simulink library "MedusaPremix"  (R2022b)
settings: Solver=VariableStepAuto  StartTime=0.0  StopTime=10.0  RelTol=1e-3
values from neighbouring files (symbols this model uses):
  PremixConfig = struct('sample_rate_in_hertz', sample_rate_in_hertz,                            'frame_size', frame_size,                            'rgain_SILENT_GAIN', rgain_SILENT_GAIN,                            'granularity', internal_granularity,                            'LR_in', LR_in, 'LR_out', LR_out,                            'CS_in', CS_in, 'CS_out', CS_out,                            'NumCenterOut' ...(+550 chars)    [MedusaPremixInit.m]
  PremixTune = MedusaPremixTuneInit(tuneFileName, headrestTuneFileName, overheadTuneFileName, MedusaParams)    [MedusaPremixInit.m]    (also in MedusaPremixTuneInit.m = load(tuneFileName))
undefined symbols (not defined in the file or in its folder): carModel, mode, MSConfig, Row
libraries: TuneVar x286, TOP x202, dspmtrx3 x146, FeaturePath x86, matrix_library x20, PooliirLib x8, Pooliir x4
(part 5 of 22)

== system MedusaPremix/PremixWithMonoSurroundAndCaeWithFadeRamper/Full Mixing Matrix_Right ==
  Audio Channel Inputs : Inport
  RST Trigger : Inport  Port=2
  SLC Request Trigger : Inport  Port=3
  In Bus Element1 : Inport  Port=4  PortName=SLC In  Element=ramp_db_per_second
  In Bus Element2 : Inport  Port=4  PortName=SLC In  Element=ramp_milliseconds
  In Bus Element : Inport  Port=4  PortName=SLC In  Element=surround_index
  SLC_NTF_check_done : Inport  Port=5
  SLC Tune In : Inport  Port=6
  Fade Request Trigger : Inport  Port=7
  Front Fade Gain : Inport  Port=8
  Back Fade Gain : Inport  Port=9
  Fade Tune In : Inport  Port=10
  Add : Sum
  Constant : Constant  OutDataTypeStr=single
  Data Store Memory1 : DataStoreMemory  DataStoreName=Premix_frameCount_Right  ReadBeforeWriteMsg=warning  WriteAfterWriteMsg=warning  WriteAfterReadMsg=warning  InitialValue=zeros(MedusaPremixConfig.LR_out,MedusaPremixConfig.LR_in)  ShowAdditionalParam=off  OutDataTypeStr=int32
  Data Store Memory2 : DataStoreMemory  DataStoreName=Premix_SLCGain_Right  ReadBeforeWriteMsg=warning  WriteAfterWriteMsg=warning  WriteAfterReadMsg=warning  InitialValue=ones(MedusaPremixConfig.LR_out,MedusaPremixConfig.LR_in)  ShowAdditionalParam=off  OutDataTypeStr=single
  Data Store Memory3 : DataStoreMemory  DataStoreName=Premix_targetGain_Right  ReadBeforeWriteMsg=warning  WriteAfterWriteMsg=warning  WriteAfterReadMsg=warning  InitialValue=ones(MedusaPremixConfig.LR_out,MedusaPremixConfig.LR_in)  ShowAdditionalParam=off  OutDataTypeStr=single
  Data Store Memory4 : DataStoreMemory  DataStoreName=Premix_currentGain_Right  ReadBeforeWriteMsg=warning  WriteAfterWriteMsg=warning  WriteAfterReadMsg=warning  InitialValue=ones(MedusaPremixConfig.LR_out,MedusaPremixConfig.LR_in)  ShowAdditionalParam=off  OutDataTypeStr=single
  Fader Downmix : Subsystem
  FeaturePath : FeaturePath/FeaturePath  FeatureName=Right  IsGroup=off  GroupNumber=-1  IsModule=off  TriggerInit=[590 34 705 141]
      settings: SourceProductName=Bose Talaria
  Matrix Multiply : Product
  Premixing : Subsystem
  Ramper : Subsystem
  Subtract : Sum  Inputs=+-
  Surround Level Control : Subsystem
  Output : Outport  VectorParamsAs1DForOutWhenUnconnected=off
  SLC_NTF_done : Outport  Port=2  VectorParamsAs1DForOutWhenUnconnected=off
  wires:
  [rampTriggerRight] -> Ramper/1(RTC Recv Trigger)
  In Bus Element1/1 -> Ramper/3(ramp rate)
  In Bus Element2/1 -> Ramper/4(ramp time)
  SLC_NTF_check_done/1 -> Ramper/5(check sequence trigger)
  [CAE_Enable] -> Fader Downmix/4(CAE_Enable)
  Front Fade Gain/1 -> Fader Downmix/1(Front Fade Gain)
  Add/1 -> Ramper/2(target gains (linear))  "Premix Matrix"
  Premixing/1(Output) -> Output/1
  Fader Downmix/2(DownmixingMatrix) -> Add/2
  SLC Tune In/1 -> Surround Level Control/4(Tuned Inputs)
  RST Trigger/1 -> Surround Level Control/1(RST Trigger)
  Ramper/1(ramping done) -> SLC_NTF_done/1
  Matrix Multiply/1 -> Add/1
  In Bus Element/1 -> Surround Level Control/3(Surround Index)
  Fade Tune In/1 -> Fader Downmix/3(Tuned Inputs)
  Fader Downmix/1(Downmix) -> Subtract/2
  Audio Channel Inputs/1 -> Premixing/1(Audio Channel Inputs)
  SLC Request Trigger/1 -> Surround Level Control/2(SLC Request Trigger)
  Fade Request Trigger/1 -> Fader Downmix/Trigger
  Back Fade Gain/1 -> Fader Downmix/2(Back Fade Gain)
  Constant/1 -> Subtract/1
  Subtract/1 -> Matrix Multiply/2  "No Downmix"
  Surround Level Control/1(Gain Out) -> Matrix Multiply/1

== system MedusaPremix/PremixWithMonoSurroundAndCaeWithFadeRamper/Generate Ramp Trigger ==
  SLCInfo : Inport
  FadeOn : Inport  Port=2
  Function-Call Split : FunctionCallSplit  IconShape=distinctive  NumOutputPorts=3  OutputPortLayout=default
  MATLAB Function : MATLAB Function  TreatAsAtomicUnit=on
  Terminator : Terminator
  tag scope: rampTriggerCS=scoped, rampTriggerLeft=scoped, rampTriggerRight=scoped
  wires:
  MATLAB Function/1(rampOn) -> Terminator/1
  SLCInfo/1 -> MATLAB Function/1(SLC_On)
  FadeOn/1 -> MATLAB Function/2(Fade_On)
  Function-Call Split/2 -> [rampTriggerCS]
  Function-Call Split/3 -> [rampTriggerRight]
  Function-Call Split/1 -> [rampTriggerLeft]
  MATLAB Function/2(ramp()) -> Function-Call Split/1

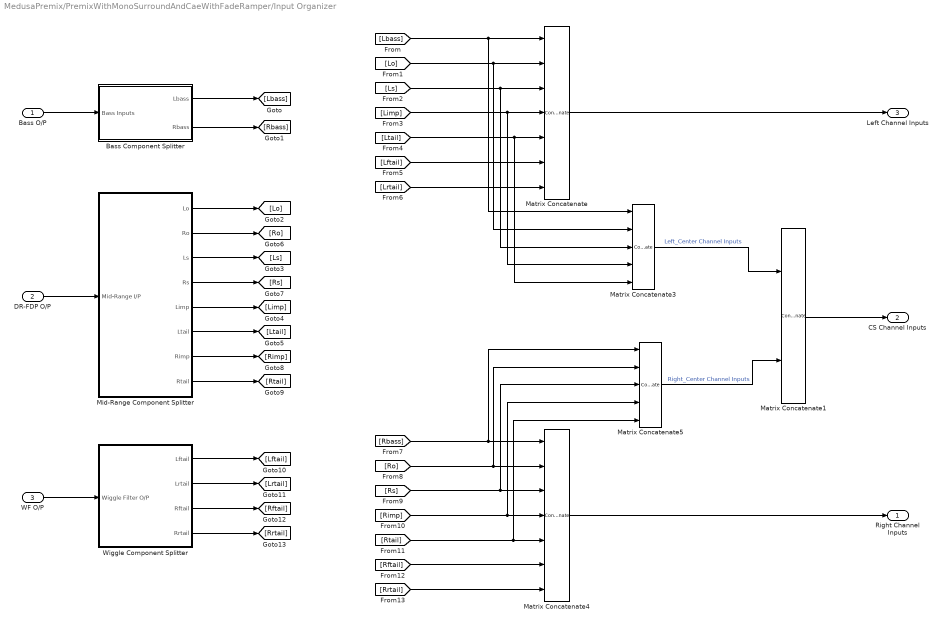
== system MedusaPremix/PremixWithMonoSurroundAndCaeWithFadeRamper/Input Organizer ==
  Bass O/P : Inport
  DR-FDP O/P : Inport  Port=2
  WF O/P : Inport  Port=3
  Bass Component Splitter : Subsystem
  Matrix Concatenate : Concatenate  NumInputs=7  Mode=Multidimensional array  ConcatenateDimension=2
  Matrix Concatenate1 : Concatenate  Mode=Multidimensional array  ConcatenateDimension=2
  Matrix Concatenate3 : Concatenate  NumInputs=5  Mode=Multidimensional array  ConcatenateDimension=2
  Matrix Concatenate4 : Concatenate  NumInputs=7  Mode=Multidimensional array  ConcatenateDimension=2
  Matrix Concatenate5 : Concatenate  NumInputs=5  Mode=Multidimensional array  ConcatenateDimension=2
  Mid-Range Component Splitter : Subsystem
  Wiggle Component Splitter : Subsystem
  Right Channel Inputs : Outport  VectorParamsAs1DForOutWhenUnconnected=off
  CS Channel Inputs : Outport  Port=2  VectorParamsAs1DForOutWhenUnconnected=off
  Left Channel Inputs : Outport  Port=3  VectorParamsAs1DForOutWhenUnconnected=off
  wires:
  Matrix Concatenate4/1 -> Right Channel Inputs/1
  [Ltail] -> Matrix Concatenate3/5, Matrix Concatenate/5
  Matrix Concatenate5/1 -> Matrix Concatenate1/2  "Right_Center Channel Inputs"
  [Limp] -> Matrix Concatenate3/4, Matrix Concatenate/4
  [Rimp] -> Matrix Concatenate5/4, Matrix Concatenate4/4
  [Rbass] -> Matrix Concatenate5/1, Matrix Concatenate4/1
  Matrix Concatenate1/1 -> CS Channel Inputs/1
  Wiggle Component Splitter/2(Lrtail) -> [Lrtail]
  Wiggle Component Splitter/1(Lftail) -> [Lftail]
  Bass Component Splitter/2(Rbass) -> [Rbass]
  DR-FDP O/P/1 -> Mid-Range Component Splitter/1(Mid-Range I/P)
  [Ro] -> Matrix Concatenate5/2, Matrix Concatenate4/2
  Wiggle Component Splitter/3(Rftail) -> [Rftail]
  Bass O/P/1 -> Bass Component Splitter/1(Bass Inputs)
  Matrix Concatenate/1 -> Left Channel Inputs/1
  [Lrtail] -> Matrix Concatenate/7
  [Lftail] -> Matrix Concatenate/6
  [Rs] -> Matrix Concatenate5/3, Matrix Concatenate4/3
  WF O/P/1 -> Wiggle Component Splitter/1(Wiggle Filter O/P)
  [Rtail] -> Matrix Concatenate5/5, Matrix Concatenate4/5
  [Ls] -> Matrix Concatenate3/3, Matrix Concatenate/3
  [Lbass] -> Matrix Concatenate3/1, Matrix Concatenate/1
  Matrix Concatenate3/1 -> Matrix Concatenate1/1  "Left_Center Channel Inputs"
  [Lo] -> Matrix Concatenate3/2, Matrix Concatenate/2
  Wiggle Component Splitter/4(Rrtail) -> [Rrtail]
  Mid-Range Component Splitter/1(Lo) -> [Lo]
  [Rftail] -> Matrix Concatenate4/6
  Bass Component Splitter/1(Lbass) -> [Lbass]
  [Rrtail] -> Matrix Concatenate4/7
  Mid-Range Component Splitter/2(Ro) -> [Ro]
  Mid-Range Component Splitter/3(Ls) -> [Ls]
  Mid-Range Component Splitter/4(Rs) -> [Rs]
  Mid-Range Component Splitter/5(Limp) -> [Limp]
  Mid-Range Component Splitter/6(Ltail) -> [Ltail]
  Mid-Range Component Splitter/7(Rimp) -> [Rimp]
  Mid-Range Component Splitter/8(Rtail) -> [Rtail]

== system MedusaPremix/PremixWithMonoSurroundAndCaeWithFadeRamper/Merge NTF_done ==
  SLC_NTF_done_Left : Inport
  SLC_NTF_done_CS : Inport  Port=2
  SLC_NTF_done_Right : Inport  Port=3
  Trigger : TriggerPort  TriggerType=function-call  VariantControl=Variant  PortDimensions=1
  AND : Logic  Inputs=3  IconShape=distinctive  AllPortsSameDT=off  OutDataTypeStr=boolean
  SLC_NTF_done : Outport  VectorParamsAs1DForOutWhenUnconnected=off
  wires:
  SLC_NTF_done_Right/1 -> AND/1
  SLC_NTF_done_CS/1 -> AND/2
  SLC_NTF_done_Left/1 -> AND/3
  AND/1 -> SLC_NTF_done/1

== system MedusaPremix/PremixWithMonoSurroundAndCaeWithFadeRamper/SLC Tuning ==
  Detent Level CS : Subsystem  Description="This is the premix (scalar mixing) matrix for the detent (default) level of \"surroundiness\"."
  Detent Level Left : Subsystem  Description="This is the premix (scalar mixing) matrix for the detent (default) level of \"surroundiness\"."
  Detent Level Right : Subsystem  Description="This is the premix (scalar mixing) matrix for the detent (default) level of \"surroundiness\"."
  Interpolation Method : Subsystem  Description=|
      | This controls the method used to interpolate premix coefficient matrix as the surround knob is adjusted.
      | - 0 for linear interpolation (default)
      | - 1 for db-linear interpolation
  Max Level CS : Subsystem  Description="This is the premix (scalar mixing) matrix for the maximum level of \"surroundiness\"."
  Max Level Left : Subsystem  Description="This is the premix (scalar mixing) matrix for the maximum level of \"surroundiness\"."
  Max Level Right : Subsystem  Description="This is the premix (scalar mixing) matrix for the maximum level of \"surroundiness\"."
  Min Level CS : Subsystem  Description="This is the premix (scalar mixing) matrix for the minimum level of \"surroundiness\" i.e. steroe case."
  Min Level Left : Subsystem  Description="This is the premix (scalar mixing) matrix for the minimum level of \"surroundiness\" i.e. steroe case."
  Min Level Right : Subsystem  Description="This is the premix (scalar mixing) matrix for the minimum level of \"surroundiness\" i.e. steroe case."
  Bus Element Out : Outport  VectorParamsAs1DForOutWhenUnconnected=off  PortName=SLC Tune Out  Element=Interpolation Method
  Bus Element Out1 : Outport  VectorParamsAs1DForOutWhenUnconnected=off  PortName=SLC Tune Out  Element=Min Level Left
  Bus Element Out2 : Outport  VectorParamsAs1DForOutWhenUnconnected=off  PortName=SLC Tune Out  Element=Detent Level Left
  Bus Element Out3 : Outport  VectorParamsAs1DForOutWhenUnconnected=off  PortName=SLC Tune Out  Element=Max Level Left
  Bus Element Out4 : Outport  VectorParamsAs1DForOutWhenUnconnected=off  PortName=SLC Tune Out  Element=Min Level CS
  Bus Element Out5 : Outport  VectorParamsAs1DForOutWhenUnconnected=off  PortName=SLC Tune Out  Element=Detent Level CS
  Bus Element Out6 : Outport  VectorParamsAs1DForOutWhenUnconnected=off  PortName=SLC Tune Out  Element=Max Level CS
  Bus Element Out7 : Outport  VectorParamsAs1DForOutWhenUnconnected=off  PortName=SLC Tune Out  Element=Min Level Right
  Bus Element Out8 : Outport  VectorParamsAs1DForOutWhenUnconnected=off  PortName=SLC Tune Out  Element=Detent Level Right
  Bus Element Out9 : Outport  VectorParamsAs1DForOutWhenUnconnected=off  PortName=SLC Tune Out  Element=Max Level Right
  Bus Element Out10 : Outport  VectorParamsAs1DForOutWhenUnconnected=off  PortName=SLC Tune Out  Element=Min Level Left CAE
  Bus Element Out11 : Outport  VectorParamsAs1DForOutWhenUnconnected=off  PortName=SLC Tune Out  Element=Detent Level Left CAE
  Bus Element Out12 : Outport  VectorParamsAs1DForOutWhenUnconnected=off  PortName=SLC Tune Out  Element=Max Level Left CAE
  Bus Element Out13 : Outport  VectorParamsAs1DForOutWhenUnconnected=off  PortName=SLC Tune Out  Element=Min Level CS CAE
  Bus Element Out14 : Outport  VectorParamsAs1DForOutWhenUnconnected=off  PortName=SLC Tune Out  Element=Detent Level CS CAE
  Bus Element Out15 : Outport  VectorParamsAs1DForOutWhenUnconnected=off  PortName=SLC Tune Out  Element=Max Level CS CAE
  Bus Element Out16 : Outport  VectorParamsAs1DForOutWhenUnconnected=off  PortName=SLC Tune Out  Element=Min Level Right CAE
  Bus Element Out17 : Outport  VectorParamsAs1DForOutWhenUnconnected=off  PortName=SLC Tune Out  Element=Detent Level Right CAE
  Bus Element Out18 : Outport  VectorParamsAs1DForOutWhenUnconnected=off  PortName=SLC Tune Out  Element=Max Level Right CAE
  wires:
  Min Level Left/2(Out2) -> Bus Element Out10/1
  Max Level Right/2(Out2) -> Bus Element Out18/1
  Detent Level Right/2(Out2) -> Bus Element Out17/1
  Min Level Right/2(Out2) -> Bus Element Out16/1
  Max Level CS/2(Out2) -> Bus Element Out15/1
  Detent Level CS/2(Out2) -> Bus Element Out14/1
  Min Level CS/2(Out2) -> Bus Element Out13/1
  Max Level Left/2(Out2) -> Bus Element Out12/1
  Detent Level Left/2(Out2) -> Bus Element Out11/1
  Min Level Right/1(Out1) -> Bus Element Out7/1
  Max Level Right/1(Out1) -> Bus Element Out9/1
  Detent Level Right/1(Out1) -> Bus Element Out8/1
  Detent Level CS/1(Out1) -> Bus Element Out5/1
  Min Level CS/1(Out1) -> Bus Element Out4/1
  Max Level CS/1(Out1) -> Bus Element Out6/1
  Max Level Left/1(Out1) -> Bus Element Out3/1
  Detent Level Left/1(Out1) -> Bus Element Out2/1
  Min Level Left/1(Out1) -> Bus Element Out1/1
  Interpolation Method/1(Out1) -> Bus Element Out/1

== system MedusaPremix/Premix/Fade Tuning/Backward Downmix Max ==
  TOP : TOP/TOP  TriggerInit=[440 20 585 80]  TopName=BackwardDownmixMax  DataType=single  BankNumber=0  Role=Automatic
      settings: SourceProductName=Bose Talaria
  TranslateTrigger : TuneVar/TranslateTrigger  TriggerInit=[286 -100 324 -45]
      settings: SourceProductName=Bose Talaria
  Trivial Translation : MATLAB Function  TreatAsAtomicUnit=on
  Tune Variable : TuneVar/Tune Variable  TuneName=BackwardDownmixMax  SpecifyMaxSize=off  VariableDim=1 (Row)  MaxSize=[1 1]  PackageName=mode  TunabilityNumber=1  MinValue=[0]  MaxValue=[1]  TriggerInit=[-65 25 105 75]  MaskValue=MedusaPremixTune.BackwardDownmixMax
      settings: SourceProductName=Bose Talaria
  Out1 : Outport  VectorParamsAs1DForOutWhenUnconnected=off
  wires:
  TOP/1 -> Out1/1  "BackwardDownmixMax"
  Tune Variable/1 -> Trivial Translation/1(BackwardDownmixMax)  "BackwardDownmixMax"
  Trivial Translation/1(TOP) -> TOP/1
  TranslateTrigger/1 -> Trivial Translation/Trigger

== system MedusaPremix/Premix/Fade Tuning/Backward Downmix Threshold ==
  TOP : TOP/TOP  TriggerInit=[440 20 585 80]  TopName=BackwardDownmixThreshold  DataType=single  BankNumber=0  Role=Automatic
      settings: SourceProductName=Bose Talaria
  TranslateTrigger : TuneVar/TranslateTrigger  TriggerInit=[306 -100 344 -45]
      settings: SourceProductName=Bose Talaria
  Trivial Translation : MATLAB Function  TreatAsAtomicUnit=on
  Tune Variable : TuneVar/Tune Variable  TuneName=BackwardDownmixThreshold  SpecifyMaxSize=off  VariableDim=1 (Row)  MaxSize=[1 1]  PackageName=mode  TunabilityNumber=1  MinValue=[0]  MaxValue=[1]  TriggerInit=[-75 25 95 75]  MaskValue=MedusaPremixTune.BackwardDownmixThreshold
      settings: SourceProductName=Bose Talaria
  Out1 : Outport  VectorParamsAs1DForOutWhenUnconnected=off
  wires:
  TOP/1 -> Out1/1  "BackwardDownmixThreshold"
  Tune Variable/1 -> Trivial Translation/1(BackwardDownmixThreshold)  "BackwardDownmixThreshold"
  Trivial Translation/1(TOP) -> TOP/1
  TranslateTrigger/1 -> Trivial Translation/Trigger

== system MedusaPremix/Premix/Fade Tuning/Downmix Weights CS ==
  TOP : TOP/TOP  TriggerInit=[440 20 585 80]  TopName=DownmixWeights_CS  DataType=single  BankNumber=0  Role=Automatic
      settings: SourceProductName=Bose Talaria
  TranslateTrigger : TuneVar/TranslateTrigger  TriggerInit=[256 -100 294 -45]
      settings: SourceProductName=Bose Talaria
  Trivial Translation : MATLAB Function  TreatAsAtomicUnit=on
  Tune Variable : TuneVar/Tune Variable  TuneName=DownmixWeights_CS  SpecifyMaxSize=off  VariableDim=1 (Row)  MaxSize=[1 1]  PackageName=mode  TunabilityNumber=1  MinValue=[0]  MaxValue=[1]  TriggerInit=[-85 25 85 75]  MaskValue=MedusaPremixTune.downmix_wts_CS
      settings: SourceProductName=Bose Talaria
  Out1 : Outport  VectorParamsAs1DForOutWhenUnconnected=off
  wires:
  TOP/1 -> Out1/1  "DownmixWeights_CS"
  Tune Variable/1 -> Trivial Translation/1(downmix_wts_CS)  "DownmixWeights_CS"
  Trivial Translation/1(TOP) -> TOP/1
  TranslateTrigger/1 -> Trivial Translation/Trigger

== system MedusaPremix/Premix/Fade Tuning/Downmix Weights Left ==
  TOP : TOP/TOP  TriggerInit=[440 20 585 80]  TopName=DownmixWeights_Left  DataType=single  BankNumber=0  Role=Automatic
      settings: SourceProductName=Bose Talaria
  TranslateTrigger : TuneVar/TranslateTrigger  TriggerInit=[266 -100 304 -45]
      settings: SourceProductName=Bose Talaria
  Trivial Translation : MATLAB Function  TreatAsAtomicUnit=on
  Tune Variable : TuneVar/Tune Variable  TuneName=DownmixWeights_Left  SpecifyMaxSize=off  VariableDim=1 (Row)  MaxSize=[1 1]  PackageName=mode  TunabilityNumber=1  MinValue=[0]  MaxValue=[1]  TriggerInit=[-80 25 90 75]  MaskValue=MedusaPremixTune.downmix_wts_Left
      settings: SourceProductName=Bose Talaria
  Out1 : Outport  VectorParamsAs1DForOutWhenUnconnected=off
  wires:
  TOP/1 -> Out1/1  "DownmixWeights_Left"
  Tune Variable/1 -> Trivial Translation/1(downmix_wts_Left)  "DownmixWeights_Left"
  Trivial Translation/1(TOP) -> TOP/1
  TranslateTrigger/1 -> Trivial Translation/Trigger

== system MedusaPremix/Premix/Fade Tuning/Downmix Weights Right ==
  TOP : TOP/TOP  TriggerInit=[475 20 620 80]  TopName=DownmixWeights_Right  DataType=single  BankNumber=0  Role=Automatic
      settings: SourceProductName=Bose Talaria
  TranslateTrigger : TuneVar/TranslateTrigger  TriggerInit=[306 -100 344 -45]
      settings: SourceProductName=Bose Talaria
  Trivial Translation : MATLAB Function  TreatAsAtomicUnit=on
  Tune Variable : TuneVar/Tune Variable  TuneName=DownmixWeights_Right  SpecifyMaxSize=off  VariableDim=1 (Row)  MaxSize=[1 1]  PackageName=mode  TunabilityNumber=1  MinValue=[0]  MaxValue=[1]  TriggerInit=[-40 25 130 75]  MaskValue=MedusaPremixTune.downmix_wts_Right
      settings: SourceProductName=Bose Talaria
  Out1 : Outport  VectorParamsAs1DForOutWhenUnconnected=off
  wires:
  TOP/1 -> Out1/1  "DownmixWeights_Right"
  Tune Variable/1 -> Trivial Translation/1(downmix_wts_Right)  "DownmixWeights_Right"
  Trivial Translation/1(TOP) -> TOP/1
  TranslateTrigger/1 -> Trivial Translation/Trigger

== system MedusaPremix/Premix/Fade Tuning/Forward Downmix Threshold ==
  TOP : TOP/TOP  TriggerInit=[440 20 585 80]  TopName=ForwardDownmixThreshold  DataType=single  BankNumber=0  Role=Automatic
      settings: SourceProductName=Bose Talaria
  TranslateTrigger : TuneVar/TranslateTrigger  TriggerInit=[291 -100 329 -45]
      settings: SourceProductName=Bose Talaria
  Trivial Translation : MATLAB Function  TreatAsAtomicUnit=on
  Tune Variable : TuneVar/Tune Variable  TuneName=ForwardDownmixThreshold  SpecifyMaxSize=off  VariableDim=1 (Row)  MaxSize=[1 1]  PackageName=mode  TunabilityNumber=1  MinValue=[0]  MaxValue=[1]  TriggerInit=[-80 25 90 75]  MaskValue=MedusaPremixTune.ForwardDownmixThreshold
      settings: SourceProductName=Bose Talaria
  Out1 : Outport  VectorParamsAs1DForOutWhenUnconnected=off
  wires:
  TOP/1 -> Out1/1  "ForwardDownmixThreshold"
  Tune Variable/1 -> Trivial Translation/1(ForwardDownmixThreshold)  "ForwardDownmixThreshold"
  Trivial Translation/1(TOP) -> TOP/1
  TranslateTrigger/1 -> Trivial Translation/Trigger

== system MedusaPremix/Premix/Fade Tuning/Foward Downmix Max ==
  TOP : TOP/TOP  TriggerInit=[440 20 585 80]  TopName=ForwardDownmixMax  DataType=single  BankNumber=0  Role=Automatic
      settings: SourceProductName=Bose Talaria
  TranslateTrigger : TuneVar/TranslateTrigger  TriggerInit=[286 -100 324 -45]
      settings: SourceProductName=Bose Talaria
  Trivial Translation : MATLAB Function  TreatAsAtomicUnit=on
  Tune Variable : TuneVar/Tune Variable  TuneName=ForwardDownmixMax  SpecifyMaxSize=off  VariableDim=1 (Row)  MaxSize=[1 1]  PackageName=mode  TunabilityNumber=1  MinValue=[0]  MaxValue=[1]  TriggerInit=[-70 25 100 75]  MaskValue=MedusaPremixTune.ForwardDownmixMax
      settings: SourceProductName=Bose Talaria
  Out1 : Outport  VectorParamsAs1DForOutWhenUnconnected=off
  wires:
  TOP/1 -> Out1/1  "ForwardDownmixMax"
  Tune Variable/1 -> Trivial Translation/1(ForwardDownmixMax)  "ForwardDownmixMax"
  Trivial Translation/1(TOP) -> TOP/1
  TranslateTrigger/1 -> Trivial Translation/Trigger

== system MedusaPremix/Premix/Full Mixing Matrix_Center Surround/Fader Downmix ==
  note: downmix
  Front Fade Gain : Inport
  Back Fade Gain : Inport  Port=2
  In Bus Element : Inport  Port=3  PortName=Tuned Inputs  Element=Forward Downmix Threshold
  In Bus Element1 : Inport  Port=3  PortName=Tuned Inputs  Element=Forward Downmix Max
  In Bus Element2 : Inport  Port=3  PortName=Tuned Inputs  Element=Backward Downmix Threshold
  In Bus Element3 : Inport  Port=3  PortName=Tuned Inputs  Element=Backward Downmix Max
  In Bus Element4 : Inport  Port=3  PortName=Tuned Inputs  Element=Downmix Weights CS
  Trigger : TriggerPort  TriggerType=function-call  VariantControl=Variant  PortDimensions=1
  Fading Backward : Subsystem  TreatAsAtomicUnit=on
  Fading Forward : Subsystem  TreatAsAtomicUnit=on
  FeaturePath : FeaturePath/FeaturePath  FeatureName=Fade  IsGroup=off  GroupNumber=-1  DeclarePackages=off  PackageNames=mode,carModel  IsToolGroup=off  TriggerInit=[920 94 1035 201]
      settings: SourceProductName=Bose Talaria
  If : If  NumInputs=2  IfExpression=u1 >= u2
  Matrix Multiply : Product
  Merge : Merge
  Downmix : Outport  VectorParamsAs1DForOutWhenUnconnected=off
  DownmixingMatrix : Outport  Port=2  VectorParamsAs1DForOutWhenUnconnected=off
  wires:
  If/1 -> Fading Forward/Action
  Fading Backward/1(downmix) -> Merge/2
  Front Fade Gain/1 -> If/1, Fading Backward/1(frontFadeGain)
  Merge/1 -> Matrix Multiply/1, Downmix/1
  Back Fade Gain/1 -> Fading Forward/1(backFadeGain), If/2
  Matrix Multiply/1 -> DownmixingMatrix/1
  Fading Forward/1(downmix) -> Merge/1
  If/2 -> Fading Backward/Action
  In Bus Element/1 -> Fading Forward/2(forwardDownmixThreshold)
  In Bus Element1/1 -> Fading Forward/3(forwardDownmixMax)
  In Bus Element2/1 -> Fading Backward/2(backwardDownmixThreshold)
  In Bus Element3/1 -> Fading Backward/3(backwardDownmixMax)
  In Bus Element4/1 -> Matrix Multiply/2

== system MedusaPremix/Premix/Full Mixing Matrix_Center Surround/Premixing ==
  Audio Channel Inputs : Inport
  Target Gain : Inport  Port=2
  Matrix Multiply1 : Product  Multiplication=Matrix(*)
  Transpose1 : Math  Operator=transpose  SignedPower=on
  Output : Outport  VectorParamsAs1DForOutWhenUnconnected=off
  wires:
  Transpose1/1 -> Matrix Multiply1/2
  Target Gain/1 -> Transpose1/1
  Audio Channel Inputs/1 -> Matrix Multiply1/1
  Matrix Multiply1/1 -> Output/1

== system MedusaPremix/Premix/Full Mixing Matrix_Center Surround/Surround Level Control ==
  RST Trigger : Inport
  SLC Request Trigger : Inport  Port=2
  In Bus Element : Inport  Port=3  PortName=Control Inputs  Element=surround_index
  In Bus Element1 : Inport  Port=3  PortName=Control Inputs  Element=ramp_db_per_second
  In Bus Element2 : Inport  Port=3  PortName=Control Inputs  Element=ramp_milliseconds
  Check Done : Inport  Port=4
  In Bus Element3 : Inport  Port=5  PortName=Tuned Inputs  Element=Min Level CS
  In Bus Element4 : Inport  Port=5  PortName=Tuned Inputs  Element=Detent Level CS
  In Bus Element5 : Inport  Port=5  PortName=Tuned Inputs  Element=Max Level CS
  In Bus Element6 : Inport  Port=5  PortName=Tuned Inputs  Element=Interpolation Method
  Data Store Memory3 : DataStoreMemory  DataStoreName=Premix_targetGain_CS  ReadBeforeWriteMsg=warning  WriteAfterWriteMsg=warning  WriteAfterReadMsg=warning  InitialValue=1e-5*ones(MedusaPremixConfig.CS_out,MedusaPremixConfig.CS_in)  ShowAdditionalParam=off  OutDataTypeStr=single
  Data Store Memory4 : DataStoreMemory  DataStoreName=Premix_currentGain_CS  ReadBeforeWriteMsg=warning  WriteAfterWriteMsg=warning  WriteAfterReadMsg=warning  InitialValue=1e-5*ones(MedusaPremixConfig.CS_out,MedusaPremixConfig.CS_in)  ShowAdditionalParam=off  OutDataTypeStr=single
  Data Store Read1 : DataStoreRead  DataStoreName=Premix_currentGain_CS  IndexOptions=Index vector (dialog)  Indices=1  OutputSizes=1
  FeaturePath : FeaturePath/FeaturePath  FeatureName=SLC  IsGroup=off  GroupNumber=-1  DeclarePackages=off  PackageNames=mode,carModel  IsToolGroup=off  TriggerInit=[955 334 1070 441]
      settings: SourceProductName=Bose Talaria
  Function-Call Split : FunctionCallSplit  IconShape=distinctive  NumOutputPorts=2
  Initialization and RMDL : MATLAB Function  TreatAsAtomicUnit=on
  Ramper : Subsystem
  Target Gain Computation : MATLAB Function  TreatAsAtomicUnit=on
  Gain Out : Outport  VectorParamsAs1DForOutWhenUnconnected=off
  Ramping Done : Outport  Port=2  VectorParamsAs1DForOutWhenUnconnected=off
  wires:
  Data Store Read1/1 -> Gain Out/1
  RST Trigger/1 -> Initialization and RMDL/Trigger
  Check Done/1 -> Ramper/5(check sequence trigger)
  Target Gain Computation/1(gain_out) -> Ramper/2(target gains (linear))
  Function-Call Split/1 -> Target Gain Computation/Trigger
  Function-Call Split/2 -> Ramper/1(RTC Recv Trigger)
  SLC Request Trigger/1 -> Function-Call Split/1
  Ramper/1(ramping done) -> Ramping Done/1
  In Bus Element5/1 -> Initialization and RMDL/3(maxGain_CS), Target Gain Computation/3(maxGain_CS)
  In Bus Element6/1 -> Initialization and RMDL/4(interpolation_method), Target Gain Computation/4(interpolation_method)
  In Bus Element3/1 -> Initialization and RMDL/1(minGain_CS), Target Gain Computation/1(minGain_CS)
  In Bus Element4/1 -> Initialization and RMDL/2(detentGain_CS), Target Gain Computation/2(detentGain_CS)
  In Bus Element2/1 -> Ramper/4(ramp time)
  In Bus Element1/1 -> Ramper/3(ramp rate)
  In Bus Element/1 -> Initialization and RMDL/5(surr_level), Target Gain Computation/5(surr_level)

== system MedusaPremix/Premix/Full Mixing Matrix_Left/Fader Downmix ==
  note: downmix
  Front Fade Gain : Inport
  Back Fade Gain : Inport  Port=2
  In Bus Element : Inport  Port=3  PortName=Tuned Inputs  Element=Forward Downmix Threshold
  In Bus Element1 : Inport  Port=3  PortName=Tuned Inputs  Element=Forward Downmix Max
  In Bus Element2 : Inport  Port=3  PortName=Tuned Inputs  Element=Backward Downmix Threshold
  In Bus Element3 : Inport  Port=3  PortName=Tuned Inputs  Element=Backward Downmix Max
  In Bus Element4 : Inport  Port=3  PortName=Tuned Inputs  Element=Downmix Weights Left
  Trigger : TriggerPort  TriggerType=function-call  VariantControl=Variant  PortDimensions=1
  Fading Backward : Subsystem  TreatAsAtomicUnit=on
  Fading Forward : Subsystem  TreatAsAtomicUnit=on
  FeaturePath : FeaturePath/FeaturePath  FeatureName=Fade  IsGroup=off  GroupNumber=-1  DeclarePackages=off  PackageNames=mode,carModel  IsToolGroup=off  TriggerInit=[875 94 990 201]
      settings: SourceProductName=Bose Talaria
  If : If  NumInputs=2  IfExpression=u1 >= u2
  Matrix Multiply : Product
  Merge : Merge
  Downmix : Outport  VectorParamsAs1DForOutWhenUnconnected=off
  DownmixingMatrix : Outport  Port=2  VectorParamsAs1DForOutWhenUnconnected=off
  wires:
  If/1 -> Fading Forward/Action
  Fading Backward/1(downmix) -> Merge/2
  Front Fade Gain/1 -> If/1, Fading Backward/1(frontFadeGain)
  Merge/1 -> Matrix Multiply/1, Downmix/1
  Back Fade Gain/1 -> Fading Forward/1(backFadeGain), If/2
  Matrix Multiply/1 -> DownmixingMatrix/1
  Fading Forward/1(downmix) -> Merge/1
  If/2 -> Fading Backward/Action
  In Bus Element/1 -> Fading Forward/2(forwardDownmixThreshold)
  In Bus Element1/1 -> Fading Forward/3(forwardDownmixMax)
  In Bus Element2/1 -> Fading Backward/2(backwardDownmixThreshold)
  In Bus Element3/1 -> Fading Backward/3(backwardDownmixMax)
  In Bus Element4/1 -> Matrix Multiply/2

== system MedusaPremix/Premix/Full Mixing Matrix_Left/Premixing ==
  Audio Channel Inputs : Inport
  Target Gain : Inport  Port=2
  Matrix Multiply1 : Product  Multiplication=Matrix(*)
  Transpose1 : Math  Operator=transpose  SignedPower=on
  Output : Outport  VectorParamsAs1DForOutWhenUnconnected=off
  wires:
  Transpose1/1 -> Matrix Multiply1/2
  Target Gain/1 -> Transpose1/1
  Audio Channel Inputs/1 -> Matrix Multiply1/1
  Matrix Multiply1/1 -> Output/1

== system MedusaPremix/Premix/Full Mixing Matrix_Left/Surround Level Control ==
  RST Trigger : Inport
  SLC Request Trigger : Inport  Port=2
  In Bus Element : Inport  Port=3  PortName=Control Inputs  Element=surround_index
  In Bus Element1 : Inport  Port=3  PortName=Control Inputs  Element=ramp_db_per_second
  In Bus Element2 : Inport  Port=3  PortName=Control Inputs  Element=ramp_milliseconds
  Check Done : Inport  Port=4
  In Bus Element3 : Inport  Port=5  PortName=Tuned Inputs  Element=Min Level Left
  In Bus Element4 : Inport  Port=5  PortName=Tuned Inputs  Element=Detent Level Left
  In Bus Element5 : Inport  Port=5  PortName=Tuned Inputs  Element=Max Level Left
  In Bus Element6 : Inport  Port=5  PortName=Tuned Inputs  Element=Interpolation Method
  Data Store Memory3 : DataStoreMemory  DataStoreName=Premix_targetGain_Left  ReadBeforeWriteMsg=warning  WriteAfterWriteMsg=warning  WriteAfterReadMsg=warning  InitialValue=1e-5*ones(MedusaPremixConfig.LR_out,MedusaPremixConfig.LR_in)  ShowAdditionalParam=off  OutDataTypeStr=single
  Data Store Memory4 : DataStoreMemory  DataStoreName=Premix_currentGain_Left  ReadBeforeWriteMsg=warning  WriteAfterWriteMsg=warning  WriteAfterReadMsg=warning  InitialValue=1e-5*ones(MedusaPremixConfig.LR_out,MedusaPremixConfig.LR_in)  ShowAdditionalParam=off  OutDataTypeStr=single
  Data Store Read1 : DataStoreRead  DataStoreName=Premix_currentGain_Left  IndexOptions=Index vector (dialog)  Indices=1  OutputSizes=1
  FeaturePath : FeaturePath/FeaturePath  FeatureName=SLC  IsGroup=off  GroupNumber=-1  DeclarePackages=off  PackageNames=mode,carModel  IsToolGroup=off  TriggerInit=[955 334 1070 441]
      settings: SourceProductName=Bose Talaria
  Function-Call Split : FunctionCallSplit  IconShape=distinctive  NumOutputPorts=2
  Initialization and RMDL : MATLAB Function  TreatAsAtomicUnit=on
  Ramper : Subsystem
  Target Gain Computation : MATLAB Function  TreatAsAtomicUnit=on
  Gain Out : Outport  VectorParamsAs1DForOutWhenUnconnected=off
  Ramping Done : Outport  Port=2  VectorParamsAs1DForOutWhenUnconnected=off
  wires:
  In Bus Element2/1 -> Ramper/4(ramp time)
  In Bus Element1/1 -> Ramper/3(ramp rate)
  In Bus Element/1 -> Target Gain Computation/5(surr_level), Initialization and RMDL/5(surr_level)
  Data Store Read1/1 -> Gain Out/1
  RST Trigger/1 -> Initialization and RMDL/Trigger
  Check Done/1 -> Ramper/5(check sequence trigger)
  Target Gain Computation/1(gain_out) -> Ramper/2(target gains (linear))
  Function-Call Split/1 -> Target Gain Computation/Trigger
  Function-Call Split/2 -> Ramper/1(RTC Recv Trigger)
  SLC Request Trigger/1 -> Function-Call Split/1
  Ramper/1(ramping done) -> Ramping Done/1
  In Bus Element5/1 -> Target Gain Computation/3(maxGain_Left), Initialization and RMDL/3(maxGain_Left)
  In Bus Element6/1 -> Target Gain Computation/4(interpolation_method), Initialization and RMDL/4(interpolation_method)
  In Bus Element3/1 -> Target Gain Computation/1(minGain_Left), Initialization and RMDL/1(minGain_Left)
  In Bus Element4/1 -> Initialization and RMDL/2(detentGain_Left), Target Gain Computation/2(detentGain_Left)

== system MedusaPremix/Premix/Full Mixing Matrix_Right/Fader Downmix ==
  note: downmix
  Front Fade Gain : Inport
  Back Fade Gain : Inport  Port=2
  In Bus Element : Inport  Port=3  PortName=Tuned Inputs  Element=Forward Downmix Threshold
  In Bus Element1 : Inport  Port=3  PortName=Tuned Inputs  Element=Forward Downmix Max
  In Bus Element2 : Inport  Port=3  PortName=Tuned Inputs  Element=Backward Downmix Threshold
  In Bus Element3 : Inport  Port=3  PortName=Tuned Inputs  Element=Backward Downmix Max
  In Bus Element4 : Inport  Port=3  PortName=Tuned Inputs  Element=Downmix Weights Right
  Trigger : TriggerPort  TriggerType=function-call  VariantControl=Variant  PortDimensions=1
  Fading Backward : Subsystem  TreatAsAtomicUnit=on
  Fading Forward : Subsystem  TreatAsAtomicUnit=on
  FeaturePath : FeaturePath/FeaturePath  FeatureName=Fade  IsGroup=off  GroupNumber=-1  DeclarePackages=off  PackageNames=mode,carModel  IsToolGroup=off  TriggerInit=[875 94 990 201]
      settings: SourceProductName=Bose Talaria
  If : If  NumInputs=2  IfExpression=u1 >= u2
  Matrix Multiply : Product
  Merge : Merge
  Downmix : Outport  VectorParamsAs1DForOutWhenUnconnected=off
  DownmixingMatrix : Outport  Port=2  VectorParamsAs1DForOutWhenUnconnected=off
  wires:
  If/1 -> Fading Forward/Action
  Fading Backward/1(downmix) -> Merge/2
  Front Fade Gain/1 -> If/1, Fading Backward/1(frontFadeGain)
  Merge/1 -> Matrix Multiply/1, Downmix/1
  Back Fade Gain/1 -> Fading Forward/1(backFadeGain), If/2
  Matrix Multiply/1 -> DownmixingMatrix/1
  Fading Forward/1(downmix) -> Merge/1
  If/2 -> Fading Backward/Action
  In Bus Element/1 -> Fading Forward/2(forwardDownmixThreshold)
  In Bus Element1/1 -> Fading Forward/3(forwardDownmixMax)
  In Bus Element2/1 -> Fading Backward/2(backwardDownmixThreshold)
  In Bus Element3/1 -> Fading Backward/3(backwardDownmixMax)
  In Bus Element4/1 -> Matrix Multiply/2

== system MedusaPremix/Premix/Full Mixing Matrix_Right/Premixing ==
  Audio Channel Inputs : Inport
  Target Gain : Inport  Port=2
  Matrix Multiply1 : Product  Multiplication=Matrix(*)
  Transpose1 : Math  Operator=transpose  SignedPower=on
  Output : Outport  VectorParamsAs1DForOutWhenUnconnected=off
  wires:
  Transpose1/1 -> Matrix Multiply1/2
  Target Gain/1 -> Transpose1/1
  Audio Channel Inputs/1 -> Matrix Multiply1/1
  Matrix Multiply1/1 -> Output/1

== system MedusaPremix/Premix/Full Mixing Matrix_Right/Surround Level Control ==
  RST Trigger : Inport
  SLC Request Trigger : Inport  Port=2
  In Bus Element : Inport  Port=3  PortName=Control Inputs  Element=surround_index
  In Bus Element1 : Inport  Port=3  PortName=Control Inputs  Element=ramp_db_per_second
  In Bus Element2 : Inport  Port=3  PortName=Control Inputs  Element=ramp_milliseconds
  Check Done : Inport  Port=4
  In Bus Element3 : Inport  Port=5  PortName=Tuned Inputs  Element=Min Level Right
  In Bus Element4 : Inport  Port=5  PortName=Tuned Inputs  Element=Detent Level Right
  In Bus Element5 : Inport  Port=5  PortName=Tuned Inputs  Element=Max Level Right
  In Bus Element7 : Inport  Port=5  PortName=Tuned Inputs  Element=Interpolation Method
  Data Store Memory3 : DataStoreMemory  DataStoreName=Premix_targetGain_Right  ReadBeforeWriteMsg=warning  WriteAfterWriteMsg=warning  WriteAfterReadMsg=warning  InitialValue=1e-5*ones(MedusaPremixConfig.LR_out,MedusaPremixConfig.LR_in)  ShowAdditionalParam=off  OutDataTypeStr=single
  Data Store Memory4 : DataStoreMemory  DataStoreName=Premix_currentGain_Right  ReadBeforeWriteMsg=warning  WriteAfterWriteMsg=warning  WriteAfterReadMsg=warning  InitialValue=1e-5*ones(MedusaPremixConfig.LR_out,MedusaPremixConfig.LR_in)  ShowAdditionalParam=off  OutDataTypeStr=single
  Data Store Read1 : DataStoreRead  DataStoreName=Premix_currentGain_Right  IndexOptions=Index vector (dialog)  Indices=1  OutputSizes=1
  FeaturePath : FeaturePath/FeaturePath  FeatureName=SLC  IsGroup=off  GroupNumber=-1  DeclarePackages=off  PackageNames=mode,carModel  IsToolGroup=off  TriggerInit=[955 334 1070 441]
      settings: SourceProductName=Bose Talaria
  Function-Call Split : FunctionCallSplit  IconShape=distinctive  NumOutputPorts=2
  Initialization and RMDL : MATLAB Function  TreatAsAtomicUnit=on
  Ramper : Subsystem
  Target Gain Computation : MATLAB Function  TreatAsAtomicUnit=on
  Gain Out : Outport  VectorParamsAs1DForOutWhenUnconnected=off
  Ramping Done : Outport  Port=2  VectorParamsAs1DForOutWhenUnconnected=off
  wires:
  Data Store Read1/1 -> Gain Out/1
  RST Trigger/1 -> Initialization and RMDL/Trigger
  Check Done/1 -> Ramper/5(check sequence trigger)
  Target Gain Computation/1(gain_out) -> Ramper/2(target gains (linear))
  Function-Call Split/1 -> Target Gain Computation/Trigger
  Function-Call Split/2 -> Ramper/1(RTC Recv Trigger)
  SLC Request Trigger/1 -> Function-Call Split/1
  Ramper/1(ramping done) -> Ramping Done/1
  In Bus Element5/1 -> Initialization and RMDL/3(maxGain_Right), Target Gain Computation/3(maxGain_Right)
  In Bus Element7/1 -> Initialization and RMDL/4(interpolation_method), Target Gain Computation/4(interpolation_method)
  In Bus Element3/1 -> Initialization and RMDL/1(minGain_Right), Target Gain Computation/1(minGain_Right)
  In Bus Element4/1 -> Initialization and RMDL/2(detentGain_Right), Target Gain Computation/2(detentGain_Right)
  In Bus Element2/1 -> Ramper/4(ramp time)
  In Bus Element1/1 -> Ramper/3(ramp rate)
  In Bus Element/1 -> Initialization and RMDL/5(surr_level), Target Gain Computation/5(surr_level)

== system MedusaPremix/Premix/Input Organizer/Bass Component Splitter ==
  Bass Inputs : Inport
  Submatrix : dspmtrx3/Submatrix  RowSpan=All rows  RowStartMode=First  RowStartIndex=1  RowEndMode=Last  RowEndIndex=1  ColSpan=One column  ColStartMode=First  ColStartIndex=1  ColEndMode=Last  ColEndIndex=1
  Submatrix1 : dspmtrx3/Submatrix  RowSpan=All rows  RowStartMode=First  RowStartIndex=1  RowEndMode=Last  RowEndIndex=1  ColSpan=One column  ColStartMode=Last  ColStartIndex=1  ColEndMode=Last  ColEndIndex=1
  Lbass : Outport  VectorParamsAs1DForOutWhenUnconnected=off
  Rbass : Outport  Port=2  VectorParamsAs1DForOutWhenUnconnected=off
  wires:
  Submatrix1/1 -> Rbass/1
  Bass Inputs/1 -> Submatrix/1, Submatrix1/1
  Submatrix/1 -> Lbass/1

== system MedusaPremix/Premix/Input Organizer/Mid-Range Component Splitter ==
  Mid-Range I/P : Inport
  Submatrix1 : dspmtrx3/Submatrix  RowSpan=All rows  RowStartMode=First  RowStartIndex=1  RowEndMode=Last  RowEndIndex=1  ColSpan=One column  ColStartMode=Index  ColStartIndex=7  ColEndMode=Last  ColEndIndex=1
  Submatrix2 : dspmtrx3/Submatrix  RowSpan=All rows  RowStartMode=First  RowStartIndex=1  RowEndMode=Last  RowEndIndex=1  ColSpan=One column  ColStartMode=Index  ColStartIndex=1  ColEndMode=Last  ColEndIndex=1
  Submatrix3 : dspmtrx3/Submatrix  RowSpan=All rows  RowStartMode=First  RowStartIndex=1  RowEndMode=Last  RowEndIndex=1  ColSpan=One column  ColStartMode=Index  ColStartIndex=2  ColEndMode=Last  ColEndIndex=1
  Submatrix4 : dspmtrx3/Submatrix  RowSpan=All rows  RowStartMode=First  RowStartIndex=1  RowEndMode=Last  RowEndIndex=1  ColSpan=One column  ColStartMode=Index  ColStartIndex=3  ColEndMode=Last  ColEndIndex=1
  Submatrix5 : dspmtrx3/Submatrix  RowSpan=All rows  RowStartMode=First  RowStartIndex=1  RowEndMode=Last  RowEndIndex=1  ColSpan=One column  ColStartMode=Index  ColStartIndex=4  ColEndMode=Last  ColEndIndex=1
  Submatrix6 : dspmtrx3/Submatrix  RowSpan=All rows  RowStartMode=First  RowStartIndex=1  RowEndMode=Last  RowEndIndex=1  ColSpan=One column  ColStartMode=Index  ColStartIndex=5  ColEndMode=Last  ColEndIndex=1
  Submatrix7 : dspmtrx3/Submatrix  RowSpan=All rows  RowStartMode=First  RowStartIndex=1  RowEndMode=Last  RowEndIndex=1  ColSpan=One column  ColStartMode=Index  ColStartIndex=6  ColEndMode=Last  ColEndIndex=1
  Submatrix8 : dspmtrx3/Submatrix  RowSpan=All rows  RowStartMode=First  RowStartIndex=1  RowEndMode=Last  RowEndIndex=1  ColSpan=One column  ColStartMode=Index  ColStartIndex=8  ColEndMode=Last  ColEndIndex=1
  Lo : Outport  VectorParamsAs1DForOutWhenUnconnected=off
  Ro : Outport  Port=2  VectorParamsAs1DForOutWhenUnconnected=off
  Ls : Outport  Port=3  VectorParamsAs1DForOutWhenUnconnected=off
  Rs : Outport  Port=4  VectorParamsAs1DForOutWhenUnconnected=off
  Limp : Outport  Port=5  VectorParamsAs1DForOutWhenUnconnected=off
  Ltail : Outport  Port=6  VectorParamsAs1DForOutWhenUnconnected=off
  Rimp : Outport  Port=7  VectorParamsAs1DForOutWhenUnconnected=off
  Rtail : Outport  Port=8  VectorParamsAs1DForOutWhenUnconnected=off
  wires:
  Submatrix3/1 -> Ro/1
  Submatrix2/1 -> Lo/1
  Submatrix4/1 -> Ls/1
  Submatrix5/1 -> Rs/1
  Submatrix7/1 -> Ltail/1
  Submatrix6/1 -> Limp/1
  Submatrix8/1 -> Rtail/1
  Submatrix1/1 -> Rimp/1
  Mid-Range I/P/1 -> Submatrix1/1, Submatrix8/1, Submatrix7/1, Submatrix2/1, Submatrix3/1, Submatrix4/1, Submatrix5/1, Submatrix6/1

== system MedusaPremix/Premix/Input Organizer/Wiggle Component Splitter ==
  Wiggle Filter O/P : Inport
  Submatrix : dspmtrx3/Submatrix  RowSpan=All rows  RowStartMode=First  RowStartIndex=1  RowEndMode=Last  RowEndIndex=1  ColSpan=One column  ColStartMode=Index  ColStartIndex=1  ColEndMode=Last  ColEndIndex=1
  Submatrix1 : dspmtrx3/Submatrix  RowSpan=All rows  RowStartMode=First  RowStartIndex=1  RowEndMode=Last  RowEndIndex=1  ColSpan=One column  ColStartMode=Index  ColStartIndex=2  ColEndMode=Last  ColEndIndex=1
  Submatrix2 : dspmtrx3/Submatrix  RowSpan=All rows  RowStartMode=First  RowStartIndex=1  RowEndMode=Last  RowEndIndex=1  ColSpan=One column  ColStartMode=Index  ColStartIndex=3  ColEndMode=Last  ColEndIndex=1
  Submatrix3 : dspmtrx3/Submatrix  RowSpan=All rows  RowStartMode=First  RowStartIndex=1  RowEndMode=Last  RowEndIndex=1  ColSpan=One column  ColStartMode=Index  ColStartIndex=4  ColEndMode=Last  ColEndIndex=1
  Lftail : Outport  VectorParamsAs1DForOutWhenUnconnected=off
  Lrtail : Outport  Port=2  VectorParamsAs1DForOutWhenUnconnected=off
  Rftail : Outport  Port=3  VectorParamsAs1DForOutWhenUnconnected=off
  Rrtail : Outport  Port=4  VectorParamsAs1DForOutWhenUnconnected=off
  wires:
  Submatrix3/1 -> Rrtail/1
  Submatrix/1 -> Lftail/1
  Wiggle Filter O/P/1 -> Submatrix3/1, Submatrix2/1, Submatrix1/1, Submatrix/1
  Submatrix2/1 -> Lrtail/1
  Submatrix1/1 -> Rftail/1

== system MedusaPremix/Premix/SLC Tuning/Detent Level CS ==
  TOP : TOP/TOP  TriggerInit=[440 20 585 80]  TopName=DetentLevel_CS  DataType=single  BankNumber=0  Role=Automatic
      settings: SourceProductName=Bose Talaria
  TranslateTrigger : TuneVar/TranslateTrigger  TriggerInit=[306 -100 344 -45]
      settings: SourceProductName=Bose Talaria
  Trivial Translation : MATLAB Function  TreatAsAtomicUnit=on
  Tune Variable : TuneVar/Tune Variable  TuneName=DetentLevel_CS  SpecifyMaxSize=off  VariableDim=1 (Row)  MaxSize=[1 1]  PackageName=mode  TunabilityNumber=1  MinValue=[0]  MaxValue=[1]  TriggerInit=[-35 25 135 75]  MaskValue=MedusaPremixTune.detentGain_CS
      settings: SourceProductName=Bose Talaria
  Out1 : Outport  VectorParamsAs1DForOutWhenUnconnected=off
  wires:
  TOP/1 -> Out1/1  "DetentLevel_CS"
  Tune Variable/1 -> Trivial Translation/1(detentGain_CS)  "DetentLevel_CS"
  Trivial Translation/1(TOP) -> TOP/1
  TranslateTrigger/1 -> Trivial Translation/Trigger

== system MedusaPremix/Premix/SLC Tuning/Detent Level Left ==
  TOP : TOP/TOP  TriggerInit=[440 20 585 80]  TopName=DetentLevel_Left  DataType=single  BankNumber=0  Role=Automatic
      settings: SourceProductName=Bose Talaria
  TranslateTrigger : TuneVar/TranslateTrigger  TriggerInit=[306 -100 344 -45]
      settings: SourceProductName=Bose Talaria
  Trivial Translation : MATLAB Function  TreatAsAtomicUnit=on
  Tune Variable : TuneVar/Tune Variable  TuneName=DetentLevel_Left  SpecifyMaxSize=off  VariableDim=1 (Row)  MaxSize=[1 1]  PackageName=mode  TunabilityNumber=1  MinValue=[0]  MaxValue=[1]  TriggerInit=[-65 25 105 75]  MaskValue=MedusaPremixTune.detentGain_Left
      settings: SourceProductName=Bose Talaria
  Out1 : Outport  VectorParamsAs1DForOutWhenUnconnected=off
  wires:
  TOP/1 -> Out1/1  "DetentLevel_Left"
  Tune Variable/1 -> Trivial Translation/1(detentGain_Left)  "DetentLevel_Left"
  Trivial Translation/1(TOP) -> TOP/1
  TranslateTrigger/1 -> Trivial Translation/Trigger

== system MedusaPremix/Premix/SLC Tuning/Detent Level Right ==
  TOP : TOP/TOP  TriggerInit=[440 20 585 80]  TopName=DetentLevel_Right  DataType=single  BankNumber=0  Role=Automatic
      settings: SourceProductName=Bose Talaria
  TranslateTrigger : TuneVar/TranslateTrigger  TriggerInit=[306 -100 344 -45]
      settings: SourceProductName=Bose Talaria
  Trivial Translation : MATLAB Function  TreatAsAtomicUnit=on
  Tune Variable : TuneVar/Tune Variable  TuneName=DetentLevel_Right  SpecifyMaxSize=off  VariableDim=1 (Row)  MaxSize=[1 1]  PackageName=mode  TunabilityNumber=1  MinValue=[0]  MaxValue=[1]  TriggerInit=[-60 25 110 75]  MaskValue=MedusaPremixTune.detentGain_Right
      settings: SourceProductName=Bose Talaria
  Out1 : Outport  VectorParamsAs1DForOutWhenUnconnected=off
  wires:
  TOP/1 -> Out1/1  "DetentLevel_Right"
  Tune Variable/1 -> Trivial Translation/1(detentGain_Right)  "DetentLevel_Right"
  Trivial Translation/1(TOP) -> TOP/1
  TranslateTrigger/1 -> Trivial Translation/Trigger

== system MedusaPremix/Premix/SLC Tuning/Interpolation Method ==
  TOP : TOP/TOP  TriggerInit=[440 20 585 80]  TopName=Interpolation_Method  DataType=single  BankNumber=0  Role=Automatic
      settings: SourceProductName=Bose Talaria
  TranslateTrigger : TuneVar/TranslateTrigger  TriggerInit=[306 -100 344 -45]
      settings: SourceProductName=Bose Talaria
  Trivial Translation : MATLAB Function  TreatAsAtomicUnit=on
  Tune Variable : TuneVar/Tune Variable  TuneName=Interpolation_Method  SpecifyMaxSize=off  VariableDim=1 (Row)  MaxSize=[1 1]  PackageName=mode  TunabilityNumber=2  MinValue=[0]  MaxValue=[1]  TriggerInit=[-40 25 130 75]  MaskValue=MedusaPremixTune.interpolationMethod
      settings: SourceProductName=Bose Talaria
  Out1 : Outport  VectorParamsAs1DForOutWhenUnconnected=off
  wires:
  TOP/1 -> Out1/1  "Interpolation_Method"
  Tune Variable/1 -> Trivial Translation/1(interpolationMethod)  "Interpolation_Method"
  Trivial Translation/1(TOP) -> TOP/1
  TranslateTrigger/1 -> Trivial Translation/Trigger

== system MedusaPremix/Premix/SLC Tuning/Max Level CS ==
  TOP : TOP/TOP  TriggerInit=[440 20 585 80]  TopName=MaxLevel_CS  DataType=single  BankNumber=0  Role=Automatic
      settings: SourceProductName=Bose Talaria
  TranslateTrigger : TuneVar/TranslateTrigger  TriggerInit=[306 -100 344 -45]
      settings: SourceProductName=Bose Talaria
  Trivial Translation : MATLAB Function  TreatAsAtomicUnit=on
  Tune Variable : TuneVar/Tune Variable  TuneName=MaxLevel_CS  SpecifyMaxSize=off  VariableDim=1 (Row)  MaxSize=[1 1]  PackageName=mode  TunabilityNumber=1  MinValue=[0]  MaxValue=[1]  TriggerInit=[-45 25 125 75]  MaskValue=MedusaPremixTune.maxGain_CS
      settings: SourceProductName=Bose Talaria
  Out1 : Outport  VectorParamsAs1DForOutWhenUnconnected=off
  wires:
  TOP/1 -> Out1/1  "MaxLevel_CS"
  Tune Variable/1 -> Trivial Translation/1(maxGain_CS)  "MaxLevel_CS"
  Trivial Translation/1(TOP) -> TOP/1
  TranslateTrigger/1 -> Trivial Translation/Trigger

== system MedusaPremix/Premix/SLC Tuning/Max Level Left ==
  TOP : TOP/TOP  TriggerInit=[440 20 585 80]  TopName=MaxLevel_Left  DataType=single  BankNumber=0  Role=Automatic
      settings: SourceProductName=Bose Talaria
  TranslateTrigger : TuneVar/TranslateTrigger  TriggerInit=[306 -100 344 -45]
      settings: SourceProductName=Bose Talaria
  Trivial Translation : MATLAB Function  TreatAsAtomicUnit=on
  Tune Variable : TuneVar/Tune Variable  TuneName=MaxLevel_Left  SpecifyMaxSize=off  VariableDim=1 (Row)  MaxSize=[1 1]  PackageName=mode  TunabilityNumber=1  MinValue=[0]  MaxValue=[1]  TriggerInit=[-55 25 115 75]  MaskValue=MedusaPremixTune.maxGain_Left
      settings: SourceProductName=Bose Talaria
  Out1 : Outport  VectorParamsAs1DForOutWhenUnconnected=off
  wires:
  TOP/1 -> Out1/1  "MaxLevel_Left"
  Tune Variable/1 -> Trivial Translation/1(maxGain_Left)  "MaxLevel_Left"
  Trivial Translation/1(TOP) -> TOP/1
  TranslateTrigger/1 -> Trivial Translation/Trigger

== system MedusaPremix/Premix/SLC Tuning/Max Level Right ==
  TOP : TOP/TOP  TriggerInit=[440 20 585 80]  TopName=MaxLevel_Right  DataType=single  BankNumber=0  Role=Automatic
      settings: SourceProductName=Bose Talaria
  TranslateTrigger : TuneVar/TranslateTrigger  TriggerInit=[306 -100 344 -45]
      settings: SourceProductName=Bose Talaria
  Trivial Translation : MATLAB Function  TreatAsAtomicUnit=on
  Tune Variable : TuneVar/Tune Variable  TuneName=MaxLevel_Right  SpecifyMaxSize=off  VariableDim=1 (Row)  MaxSize=[1 1]  PackageName=mode  TunabilityNumber=1  MinValue=[0]  MaxValue=[1]  TriggerInit=[-40 25 130 75]  MaskValue=MedusaPremixTune.maxGain_Right
      settings: SourceProductName=Bose Talaria
  Out1 : Outport  VectorParamsAs1DForOutWhenUnconnected=off
  wires:
  TOP/1 -> Out1/1  "MaxLevel_Right"
  Tune Variable/1 -> Trivial Translation/1(maxGain_Right)  "MaxLevel_Right"
  Trivial Translation/1(TOP) -> TOP/1
  TranslateTrigger/1 -> Trivial Translation/Trigger

== system MedusaPremix/Premix/SLC Tuning/Min Level CS ==
  TOP : TOP/TOP  TriggerInit=[440 20 585 80]  TopName=MinLevel_CS  DataType=single  BankNumber=0  Role=Automatic
      settings: SourceProductName=Bose Talaria
  TranslateTrigger : TuneVar/TranslateTrigger  TriggerInit=[306 -100 344 -45]
      settings: SourceProductName=Bose Talaria
  Trivial Translation : MATLAB Function  TreatAsAtomicUnit=on
  Tune Variable : TuneVar/Tune Variable  TuneName=MinLevel_CS  SpecifyMaxSize=off  VariableDim=1 (Row)  MaxSize=[1 1]  PackageName=mode  TunabilityNumber=1  MinValue=[0]  MaxValue=[1]  TriggerInit=[-45 25 125 75]  MaskValue=MedusaPremixTune.minGain_CS
      settings: SourceProductName=Bose Talaria
  Out1 : Outport  VectorParamsAs1DForOutWhenUnconnected=off
  wires:
  TOP/1 -> Out1/1  "MinLevel_CS"
  Tune Variable/1 -> Trivial Translation/1(minGain_CS)  "MinLevel_CS"
  Trivial Translation/1(TOP) -> TOP/1
  TranslateTrigger/1 -> Trivial Translation/Trigger
